simulink model "foc_speedcontroller"  (R2026a)
settings: Solver=FixedStepDiscrete  FixedStep=foc.Ts*10
undefined symbols (not defined in the file): foc, pmsm
libraries: mcbcontrollergainlib x1, slpidlib x1
settings Model: Creator=probst  LastModifiedBy=probst

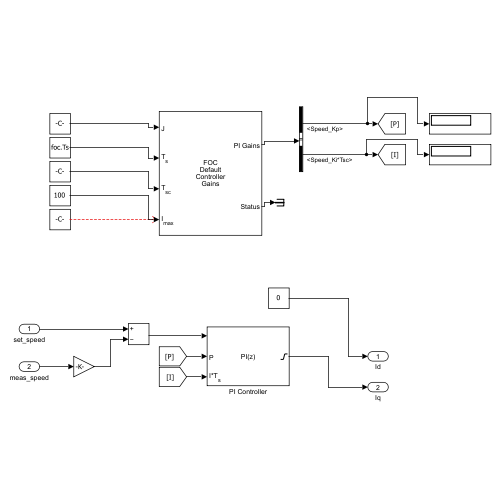
[thumbnail: Simulink's stored preview of the top-level diagram]
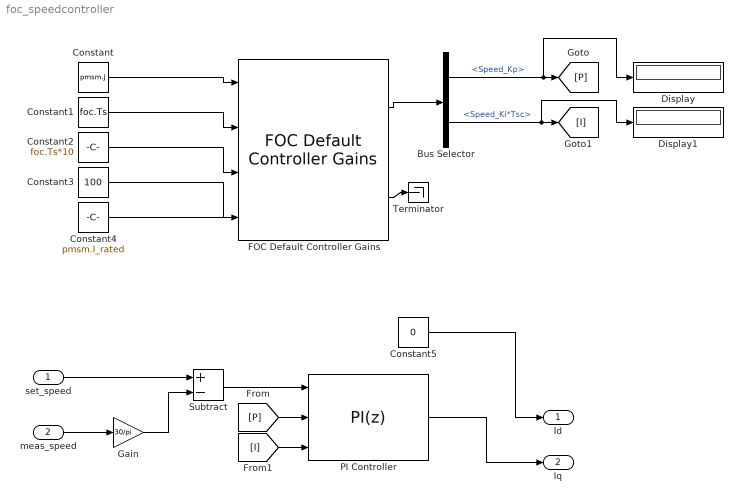
== system foc_speedcontroller ==
  set_speed : Inport
  meas_speed : Inport  Port=2
  Bus Selector : BusSelector  OutputSignals=Speed_Kp,Speed_Ki*Tsc
  Constant : Constant  Value=pmsm.J
  Constant1 : Constant  Value=foc.Ts
  Constant2 : Constant  Value=foc.Ts*10
  Constant3 : Constant  Value=100
  Constant4 : Constant  Value=pmsm.I_rated
  Constant5 : Constant  Value=0
  Display : Display
  Display1 : Display
  FOC Default Controller Gains : mcbcontrollergainlib/FOC Default Controller Gains  ControllerGainType=Empirical method  motorSelection=PMSM  unitType=SI Unit  EnObserver=off  ObsType=Flux Observer (Only for SPMSM)  ObsCutOffFrq=10  outCurrentControlGain=off  outFWCGain=off  outSpeedControlGain=on  externalDelay=on  currentSensorDelay=Ts  speedSensorDelay=Ts  speedFilterDelay=0
      settings: LibrarySourceBlock=mcblib/Controls/Controllers/FOC Default Controller Gains
  Gain : Gain  Gain=30/pi
  PI Controller : slpidlib/PID Controller  Controller=PI  Form=Parallel  TimeDomain=Discrete-time  UseExternalTs=off  SampleTime=-1  IntegratorMethod=Forward Euler  FilterMethod=Forward Euler  ControllerParametersSource=external  P=1  I=1  UseKiTs=on  D=0  UseExternalDerivativeSource=off  N=100  UseFilter=on  TunerSelectOption=Transfer Function Based (PID Tuner App)  InitialConditionSource=internal  InitialConditionForIntegrator=0  InitialConditionForFilter=0  DifferentiatorICPrevScaledInput=0  ExternalReset=none  TrackingMode=off  Kt=1  LimitOutput=on  SatLimitsSource=internal  UpperSaturationLimit=pmsm.I_rated  LowerSaturationLimit=-pmsm.I_rated  LinearizeAsGain=on  AntiWindupMode=clamping  Kb=1  LimitIntegrator=on  UpperIntegratorSaturationLimit=pmsm.I_rated  LowerIntegratorSaturationLimit=-pmsm.I_rated  RndMeth=Simplest  POutMin=[]  POutMax=[]  IOutMin=[]  IOutMax=[]  DOutMin=[]  DOutMax=[]  NOutMin=[]  NOutMax=[]  SumOutMin=[]  SumOutMax=[]  SaturationOutDataTypeStr=Inherit: Inherit via back propagation  SaturationOutMin=[]  SaturationOutMax=[]  PParamMin=[]  PParamMax=[]  IParamMin=[]  IParamMax=[]  DParamMin=[]  DParamMax=[]  NParamMin=[]  NParamMax=[]  KbParamMin=[]  KbParamMax=[]  KtParamMin=[]  KtParamMax=[]  KbOutMin=[]  KbOutMax=[]  KtOutMin=[]  KtOutMax=[]  IntegratorOutMin=[]  IntegratorOutMax=[]  FilterOutMin=[]  FilterOutMax=[]  SumI1OutMin=[]  SumI1OutMax=[]  SumI2OutMin=[]  SumI2OutMax=[]  SumI3OutMin=[]  SumI3OutMax=[]  SumI4OutMin=[]  SumI4OutMax=[]  SumDOutMin=[]  SumDOutMax=[]  DifferentiatorOutMin=[]  DifferentiatorOutMax=[]  FilterDiffOutCoefMin=[]  FilterDiffOutCoefMax=[]  ReciprocalOutMin=[]  ReciprocalOutMax=[]  SumDenOutMin=[]  SumDenOutMax=[]  SumNumOutMin=[]  SumNumOutMax=[]  DivideOutMin=[]  DivideOutMax=[]  UdiffTsProdOutMin=[]  UdiffTsProdOutMax=[]  NTsProdOutMin=[]  NTsProdOutMax=[]  UintegralTsProdOutMin=[]  UintegralTsProdOutMax=[]  UngainTsProdOutMin=[]  UngainTsProdOutMax=[]  ClampingZeroOutDataTypeStr=Inherit: Inherit via back propagation  ClampingZeroOutMin=[]  ClampingZeroOutMax=[]  FilterDenConstantOutDataTypeStr=Inherit: Inherit via back propagation  FilterDenConstantOutMin=[]  FilterDenConstantOutMax=[]  PCopyOutDataTypeStr=Inherit: Inherit via back propagation  PCopyOutMin=[]  PCopyOutMax=[]  NCopyOutDataTypeStr=Inherit: Inherit via back propagation  NCopyOutMin=[]  NCopyOutMax=[]  IntegratorContinuousStateAttributes=''  IntegratorStateMustResolveToSignalObject=off  IntegratorRTWStateStorageClass=Auto  FilterContinuousStateAttributes=''  FilterStateMustResolveToSignalObject=off  FilterRTWStateStorageClass=Auto  ParallelPVariant=ExternalParameters  IdealPVariant=Disabled  IVariant=ExternalParameters  DVariant=Disabled  IntegratorVariant=Discrete  SatVariant=Enabled  AWVariant=DiscClampingParallel  PCopyVariant=Disabled  TRVariant=Disabled  FdbkBlocksVariant=Forward  IdealPFdbkVariant=Disabled  SatFdbkVariant=Disabled  DerivativeFilterVariant=Disabled  NVariant=Disabled  NCopyVariant=Disabled_SignalSpec  FilterICVariant=Disabled  IntegratorICVariant=InternalICs  ExternalResetVariant=Disabled  TRSumVariant=Passthrough  SumFdbkVariant=Disabled  SumVariant=Sum_PI  TsampFilterVariant=InternalTs  TsampNgainVariant=Passthrough  TsampIntegralVariant=Disabled_SignalSpec  ExternalSaturationOutDataTypeStr=Inherit: Same as second input  DerivativeSourceVariant=Disabled  PreIntVariant=InternalPreInt
      settings: LibrarySourceBlock=mcblib/Controls/Controllers/PI Controller
  Subtract : Sum  Inputs=+-
  Terminator : Terminator
  Id : Outport
  Iq : Outport  Port=2
  wires:
  set_speed/1 -> Subtract/1
  Subtract/1 -> PI Controller/1
  meas_speed/1 -> Gain/1
  [P] -> PI Controller/2
  [I] -> PI Controller/3
  FOC Default Controller Gains/1 -> Bus Selector/1
  Bus Selector/1 -> Display/1, [P]  "<Speed_Kp>"
  Bus Selector/2 -> Display1/1, [I]  "<Speed_Ki*Tsc>"
  FOC Default Controller Gains/2 -> Terminator/1
  Constant/1 -> FOC Default Controller Gains/1
  Constant1/1 -> FOC Default Controller Gains/2
  Constant2/1 -> FOC Default Controller Gains/3
  Constant4/1 -> ?
  Constant3/1 -> FOC Default Controller Gains/4
  PI Controller/1 -> Iq/1
  Constant5/1 -> Id/1
  Gain/1 -> Subtract/2
